simulink model "Copy_3_of_soft_switch_new_simulation"  (R2025b)
settings: Solver=ode23s  StartTime=0.0  StopTime=1  MaxStep=1e-6  RelTol=1e-5
InitFcn:
  | run param_file.m
values from neighbouring files (symbols this model uses):
  param = struct()    [Copy_of_param_file.m]    (also in param_file.m; param_file_loss_vs_freq.m; param_file_original.m; param_file_turbine.m)
settings Model: Creator=user  LastModifiedBy=user
settings SolverCC: ZeroCrossAlgorithm=Adaptive
settings DebuggingCC: IgnoredZcDiagnostic=none

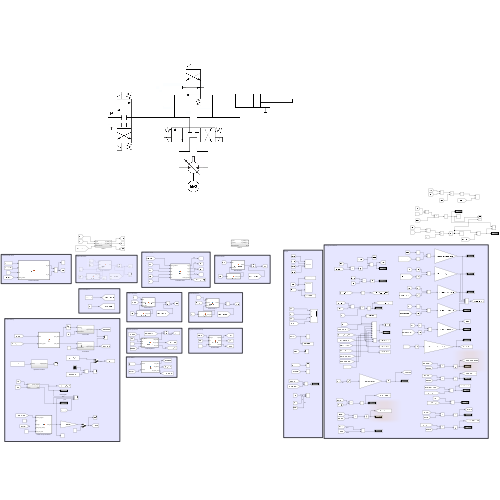
[thumbnail: Simulink's stored preview of the top-level diagram]
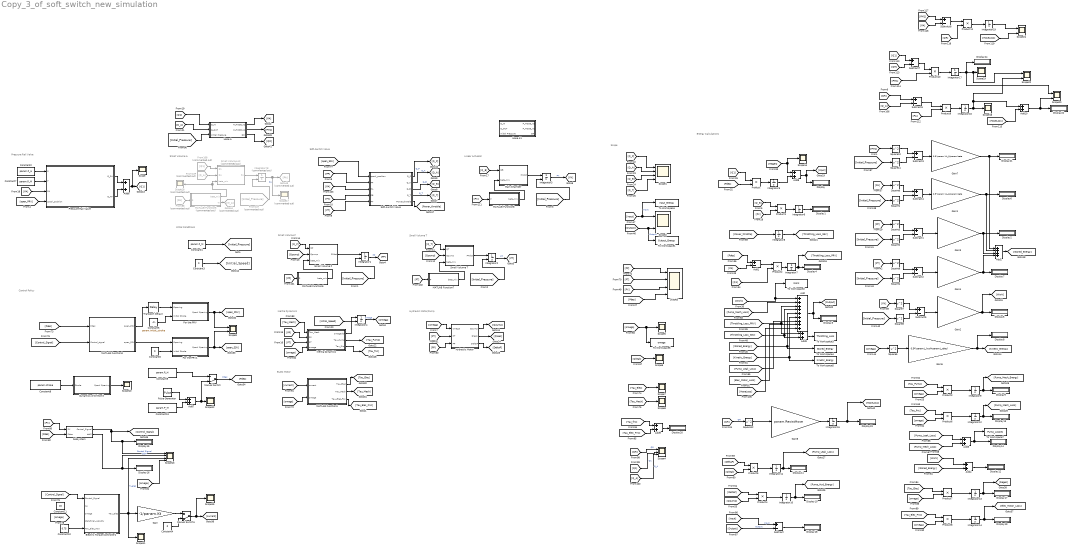
== system Copy_3_of_soft_switch_new_simulation ==
  note: Small Volume A
  note: Control Policy
  note: BLDC Motor
  note: Energy Calculations
  note: Pressure Rail Valve
  note: Scope
  note: Initial Conditions
  note: Hydraulic Motor/Pump
  note: Inertia Dynamics
  note: Small Volume T
  note: Small Volume P
  note: Soft-Switch Valve
  note: Linear Actuator
  Add : Sum  Inputs=+++++++++
  Add1 : Sum  Inputs=+-
  Add{3..10} (8 alike) : Sum
  Add2 : Sum  Inputs=++++
  Constant1 : Constant  Value=param.P_M
  Constant10 : Constant  Value=0.75
  Constant11 : Constant  Value=15
  Constant13 : Constant  Value=param.P_M
  Constant2 : Constant  Value=param.P_H
  Constant3 : Constant  Value=0
  Constant4 : Constant  Value=0
  Constant5 : Constant  Value=param.initial_stroke
  Constant6 : Constant  Value=0
  Constant7 : Constant  Value=param.P_M
  Constant8 : Constant  Value=param.stroke
  Constant9 : Constant  Value=param.P_H
  Display{,1..24} (25 alike) : Display
  Dynamics of Orifice 3 : Subsystem
  Electric Torque Controller1 : MATLAB Function  TreatAsAtomicUnit=on
  For the PRV : Subsystem
  For the PRV1 : Subsystem
  From107 : From  Commented=on  GotoTag=Initial_Pressure
  From108 : From  Commented=on  GotoTag=Q1
  From109 : From  Commented=on  GotoTag=Q_A
  From88 : From  Commented=on  GotoTag=PA
  Gain : Gain  Gain=-1/param.Kt
  Gain1 : Gain  Gain=0.5*param.VA_0/param.beta
  Gain2 : Gain  Gain=0.5*param.V1_0/param.beta
  Gain3 : Gain  Gain=0.5*param.VP_0/param.beta
  Gain4 : Gain  Gain=0.5*param.VT_0/param.beta
  Gain5 : Gain  Gain=0.5*(param.J_hyd+param.J_elec)
  Gain7 : Gain  Gain=0.5*param.VA_0/param.beta
  Gain8 : Gain  Gain=param.ResistHose
  Goto43 : Goto  Commented=on  GotoTag=PA
  Goto44 : Goto  Commented=on  GotoTag=W_A
  Hose A : Subsystem
  Hose A1 : Subsystem
  Hydraulic Motor : MATLAB Function  TreatAsAtomicUnit=on
  Inertia Dynamics : MATLAB Function  TreatAsAtomicUnit=on
  Integrator{1..4} (4 alike) : Integrator  InitialConditionSource=external
  Integrator{5..17,19} (14 alike) : Integrator
  Integrator18 : Integrator  Commented=on  InitialConditionSource=external
  MATLAB Function1 : MATLAB Function  TreatAsAtomicUnit=on
  MATLAB Function3 : MATLAB Function  TreatAsAtomicUnit=on
  MATLAB Function5 : MATLAB Function  Commented=on  TreatAsAtomicUnit=on
  MATLAB Function6 : MATLAB Function  TreatAsAtomicUnit=on
  MATLAB Function7 : MATLAB Function  TreatAsAtomicUnit=on
  MATLAB Function8 : MATLAB Function  TreatAsAtomicUnit=on
  Main Chamber : MATLAB Function  TreatAsAtomicUnit=on
  Manual Switch : ManualSwitch  CurrentSetting=0
  Manual Switch1 : ManualSwitch  CurrentSetting=0
  Pressure Rail Valve : MATLAB Function  TreatAsAtomicUnit=on
  Product{,1..11} (12 alike) : Product
  Pulse Generator : DiscretePulseGenerator  PulseType=Time based  Amplitude=param.P_H-param.P_M  Period=1.0  PulseWidth=50  PhaseDelay=param.delay
  Scope{,5..8,10..12,14..16,19} (12 alike) : Scope
      Scope settings: ActiveDisplayYMinimum=-7.8990948168927051E-6  ActiveDisplayYMaximum=6.46174239346027E-5  DataLoggingVariableName=ScopeData14
      Scope10 settings: ActiveDisplayYMinimum=-0.00062  ActiveDisplayYMaximum=0.00562  DataLoggingVariableName=ScopeData9
      Scope11 settings: ActiveDisplayYMinimum=-0.9375  ActiveDisplayYMaximum=0.9375  DataLoggingVariableName=ScopeData10
      Scope12 settings: ActiveDisplayYMinimum=2.585125E+6  ActiveDisplayYMaximum=1.1203875E+7  DataLoggingVariableName=ScopeData11
      Scope14 settings: ActiveDisplayYMinimum=-0.0475518283401892  ActiveDisplayYMaximum=0.42796645506170294  DataLoggingVariableName=ScopeData13
      Scope15 settings: ActiveDisplayYMinimum=-1  ActiveDisplayYMaximum=1  DataLoggingVariableName=ScopeData15
      Scope16 settings: ActiveDisplayYMinimum=-0.0475518283401892  ActiveDisplayYMaximum=0.42796645506170294  DataLoggingVariableName=ScopeData16
      Scope19 settings: ActiveDisplayYMinimum=-0.0475518283401892  ActiveDisplayYMaximum=0.42796645506170294  DataLoggingVariableName=ScopeData19
      Scope5 settings: ActiveDisplayYMinimum=-11.518295379628592  ActiveDisplayYMaximum=103.66465841665735  DataLoggingVariableName=ScopeData3
      Scope6 settings: ActiveDisplayYMinimum=-2.1163885820684094E-7  ActiveDisplayYMaximum=1.4152197079471591E-6  DataLoggingVariableName=ScopeData5
      Scope7 settings: ActiveDisplayYMinimum=-0.75527710182478136  ActiveDisplayYMaximum=-0.74781146844223478  DataLoggingVariableName=ScopeData6
      Scope8 settings: ActiveDisplayYMinimum=-0.030512320140982374  ActiveDisplayYMaximum=0.010920175405050834  DataLoggingVariableName=ScopeData7
  Scope1 : Scope  NumInputPorts=4
      settings: ActiveDisplayYMinimum=-0.00094060960760663083  ActiveDisplayYMaximum=0.00094060960760663083
  Scope13 : Scope  NumInputPorts=4
      settings: ActiveDisplayYMinimum=-0.12499999999999997  ActiveDisplayYMaximum=1.125  DataLoggingVariableName=ScopeData12
  Scope17 : Scope  Commented=on
      settings: ActiveDisplayYMinimum=2.181490968537122E+6  ActiveDisplayYMaximum=1.1231186415855616E+7  DataLoggingVariableName=ScopeData17
  Scope18 : Scope  Commented=on
      settings: ActiveDisplayYMinimum=1.7999999999999995E+9  ActiveDisplayYMaximum=1.8000000000000005E+9  DataLoggingVariableName=ScopeData18
  Scope{2,9,20..22} (5 alike) : Scope  NumInputPorts=2
      Scope2 settings: ActiveDisplayYMinimum=7.1801109176993929  ActiveDisplayYMaximum=9.674075574850372
      Scope20 settings: ActiveDisplayYMinimum=-0.032471059500060594  ActiveDisplayYMaximum=0.29223953550054538  DataLoggingVariableName=ScopeData20
      Scope21 settings: ActiveDisplayYMinimum=0.0065545365795663139  ActiveDisplayYMaximum=0.0079304272883429627  DataLoggingVariableName=ScopeData21
      Scope22 settings: ActiveDisplayYMinimum=-0.033093611834101345  ActiveDisplayYMaximum=0.29784250650691219  DataLoggingVariableName=ScopeData22
      Scope9 settings: ActiveDisplayYMinimum=-1.2499999999999898  ActiveDisplayYMaximum=1.2499999999999079  DataLoggingVariableName=ScopeData8
  Scope3 : Scope  NumInputPorts=4
      settings: ActiveDisplayYMinimum=-38180.936985161854  ActiveDisplayYMaximum=1.3423951077997142E+7  DataLoggingVariableName=ScopeData2
  Scope4 : Scope  NumInputPorts=3
      settings: ActiveDisplayYMinimum=-1.8027015658563681E-5  ActiveDisplayYMaximum=0.00016224314092707316  DataLoggingVariableName=ScopeData4
  Small Volume A2 : MATLAB Function  Commented=on  TreatAsAtomicUnit=on
  Small Volume P : MATLAB Function  TreatAsAtomicUnit=on
  Small Volume T : MATLAB Function  TreatAsAtomicUnit=on
  Soft-switch Valve : MATLAB Function  TreatAsAtomicUnit=on
  Square{1..12} (12 alike) : Math  Operator=square
  Subsystem : Subsystem
  Subtract{,1..8} (9 alike) : Sum  Inputs=+-
  To Workspace : ToWorkspace  VariableName=Input_Energy  SaveFormat=Timeseries  SampleTime=-1
  To Workspace1 : ToWorkspace  VariableName=Output_Energy  SaveFormat=Timeseries  SampleTime=-1
  To Workspace2 : ToWorkspace  VariableName=Work  SaveFormat=Timeseries  SampleTime=-1
  To Workspace3 : ToWorkspace  VariableName=Throttling_Loss  SaveFormat=Timeseries  SampleTime=-1
  To Workspace4 : ToWorkspace  VariableName=Stored_Energy  SaveFormat=Timeseries  SampleTime=-1
  To Workspace5 : ToWorkspace  VariableName=Kinetic_Energy  SaveFormat=Timeseries  SampleTime=-1
  To Workspace6 : ToWorkspace  VariableName=omega  SaveFormat=Timeseries  SampleTime=-1
  To Workspace7 : ToWorkspace  VariableName=Pump_Losses  SaveFormat=Timeseries  SampleTime=-1
  Transport Delay2 : TransportDelay  DelayTime=10e-3  InitialOutput=param.initial_stroke  BufferSize=1024*105
  wires:
  Constant2/1 -> Pressure Rail Valve/1(P)
  Constant1/1 -> [Initial_Pressure]
  Small Volume P/1(PPdot) -> Integrator1/1
  [Initial_Pressure] -> Integrator1/2
  Small Volume T/1(PTdot) -> Integrator2/1
  [Initial_Pressure] -> Integrator2/2
  Main Chamber/1(PXdot) -> Integrator3/1
  [Initial_Pressure] -> Integrator3/2
  Integrator3/1 -> [PX]  "PX"
  [PA] -> Soft-switch Valve/3(PA)
  [omega] -> Hydraulic Motor/1(omega)
  Integrator1/1 -> [PP]  "PP"
  Integrator2/1 -> [PT]  "PT"
  [PP] -> Soft-switch Valve/2(PP)
  [PT] -> Soft-switch Valve/5(PT)
  [PX] -> Soft-switch Valve/4(PB)
  Soft-switch Valve/4(Q_T) -> [Q_T]  "Q_T"
  Soft-switch Valve/3(Q_B) -> [Q_B]  "Q_B"
  Soft-switch Valve/2(Q_A) -> [Q_A]  "Q_A"
  [Q_T] -> Small Volume T/1(QT)
  Hydraulic Motor/1(Qpump) -> [Qpump]
  [Qpump] -> Small Volume T/2(Qpump)
  [Qpump] -> Small Volume P/2(Qpump)
  [Q_P] -> Small Volume P/1(QP)
  [Q_B] -> Main Chamber/1(QB)
  Constant3/1 -> [Initial_Speed]
  [Q_P] -> Scope1/1
  [Q_A] -> Scope1/2
  [Q_B] -> Scope1/3
  [Q_T] -> Scope1/4
  [Q1] -> Product/1
  [Pdes] -> Product/2
  Product/1 -> Integrator5/1
  [Q_B] -> Product1/1
  [PX] -> Product1/2
  Product1/1 -> Integrator6/1
  Integrator6/1 -> Display1/1
  [Work] -> To Workspace2/1, Add/1
  [Kinetic_Energy] -> To Workspace5/1, Add/6
  Add/1 -> [Output], Display3/1
  [PA] -> Add1/2
  Add1/1 -> Product2/1
  [Q1] -> Product2/2
  Product2/1 -> Integrator7/1
  Integrator7/1 -> [Throttling_Loss_PRV], Display4/1
  [Throttling_Loss_PRV] -> Add3/1, Add/3
  Soft-switch Valve/1(Q_P) -> [Q_P]  "Q_P"
  Soft-switch Valve/5(Power_throttle) -> [Power_throttle]
  [PA] -> Square6/1
  Subtract5/1 -> Gain2/1
  Gain2/1 -> [Work], Display5/1
  Gain1/1 -> Add2/2, Display6/1
  Gain3/1 -> Add2/3, Display2/1
  Gain5/1 -> Display8/1, [Kinetic_Energy]
  Square5/1 -> Gain5/1
  [omega] -> Square5/1
  [Stored_Energy] -> To Workspace4/1, Add/5
  [Initial_Pressure] -> Square1/1
  Square6/1 -> Subtract4/1
  Square1/1 -> Subtract4/2
  [PX] -> Square7/1
  [Initial_Pressure] -> Square8/1
  Subtract4/1 -> Gain1/1
  Square7/1 -> Subtract5/1
  Square8/1 -> Subtract5/2
  Square2/1 -> Subtract1/2
  Square3/1 -> Subtract1/1
  Square9/1 -> Subtract2/1
  Square4/1 -> Subtract2/2
  Subtract2/1 -> Gain4/1
  [PT] -> Square9/1
  [Initial_Pressure] -> Square4/1
  [PP] -> Square3/1
  [Initial_Pressure] -> Square2/1
  Subtract1/1 -> Gain3/1
  Gain4/1 -> Add2/4, Display7/1
  Add2/1 -> [Stored_Energy]
  [Input] -> Scope2/1, To Workspace/1  "Input"
  [Output] -> To Workspace1/1, Scope2/2  "Output"
  Integrator8/1 -> [Throttling_Loss_SSV]
  [Throttling_Loss_SSV] -> Add3/2, Add/4
  Add3/1 -> To Workspace3/1
  [PX] -> Scope3/3
  [PT] -> Inertia Dynamics/3(PT)
  Inertia Dynamics/2(Tau_Pump) -> [Tau_Pump]
  [PP] -> Inertia Dynamics/2(PP)
  [omega] -> Product3/2
  [Tau_Pump] -> Product3/1
  Integrator9/1 -> [Pump_Mech_Energy], Display9/1
  Product3/1 -> Integrator9/1
  Hydraulic Motor/3(DeltaP) -> [DeltaP]
  [DeltaP] -> Product4/1
  [Qpump] -> Product4/2
  Product4/1 -> Integrator10/1
  Integrator10/1 -> [Pump_Hyd_Energy], Display10/1
  [omega] -> To Workspace6/1, Scope5/1
  Hydraulic Motor/2(Qleak) -> [Qleak]
  [Qleak] -> Scope6/1
  [PT] -> Hydraulic Motor/2(PT)
  [PP] -> Hydraulic Motor/3(PP)
  [DeltaP] -> Product5/1
  [Qleak] -> Product5/2
  Product5/1 -> Integrator11/1
  Integrator11/1 -> [Pump_Leak_Loss], Display11/1
  [Pump_Mech_Loss] -> Add/2
  [omega] -> Inertia Dynamics/4(omega)
  Inertia Dynamics/3(Tau_Fric) -> [Tau_fric]
  [Tau_fric] -> Product6/1
  [omega] -> Product6/2
  Product6/1 -> Integrator12/1
  Integrator12/1 -> [Pump_Mech_Loss], Display13/1
  [Pump_Leak_Loss] -> Add/7
  [Pump_Leak_Loss] -> Add5/1
  [Pump_Mech_Loss] -> Add5/2
  Add5/1 -> To Workspace7/1, Display14/1
  [Work] -> Add4/1
  [Stored_Energy] -> Add4/2
  Add4/1 -> Display12/1
  [Pdes] -> Scope3/4
  [PT] -> Scope3/2
  [PP] -> Scope3/1
  [omega] -> MATLAB Function1/2(omega)
  [current] -> MATLAB Function1/1(current)
  MATLAB Function1/1(Tau_Elec) -> [Tau_Elec]
  MATLAB Function1/2(Tau_Mech) -> [Tau_Mech]
  [Tau_Elec] -> Scope7/1
  [Tau_Mech] -> Scope8/1
  For the PRV/1(Spool Opening) -> [open_PRV], Scope9/1
  For the PRV1/1(Spool Opening) -> Scope9/2, [open_SSV]
  [Control_Signal] -> MATLAB Function3/2(Control_signal)
  Transport Delay2/1 -> For the PRV/1(Opening)
  MATLAB Function3/1(open_PRV) -> Transport Delay2/1
  MATLAB Function3/2(open_SSV) -> For the PRV1/1(Opening)
  Pressure Rail Valve/1(Q_PA) -> Add6/1
  Pressure Rail Valve/2(Q_AT) -> Add6/2
  Add6/1 -> Scope/1, [Q1]
  [PA] -> Pressure Rail Valve/3(PA)
  Constant7/1 -> Pressure Rail Valve/2(T)
  [open_PRV] -> Pressure Rail Valve/4(spool_position)
  [open_SSV] -> Soft-switch Valve/1(spool_position)
  [Pdes] -> Subsystem/2(Pdes)
  [PX] -> Subsystem/1(PX)
  Subsystem/1(Control_Signal) -> [Control_Signal], Scope13/1, Display15/1  "Control Signal"
  Subsystem/2(delP) -> Scope13/2, Display16/1  "delP"
  Manual Switch/1 -> [Pdes]  "Pdes"
  Constant10/1 -> Electric Torque Controller1/5(Tau_elec_max)
  Constant9/1 -> Manual Switch/1
  Constant13/1 -> Add7/2
  Pulse Generator/1 -> Add7/1
  Add7/1 -> Manual Switch/2, Scope12/1
  Dynamics of Orifice 3/1(Spool Opening) -> Scope10/1
  Constant8/1 -> Dynamics of Orifice 3/1(Stroke)
  [omega] -> Scope13/4
  [Control_Signal] -> Electric Torque Controller1/1(Control_Signal)
  Electric Torque Controller1/1(Tau_elec) -> Gain/1, Scope13/3, Scope11/1  "T_elec"
  [Pdes] -> MATLAB Function3/1(Pdes)
  [Tau_Elec] -> Product7/1
  [omega] -> Product7/2
  Product7/1 -> Integrator13/1
  Integrator13/1 -> [Regen], Display17/1
  [Input] -> Subtract/1  "Input"
  [Output] -> Subtract/2  "Output"
  Subtract/1 -> Display18/1
  MATLAB Function1/3(Tau_Elec_Fric) -> [Tau_Elec_Fric]
  [Tau_Elec_Fric] -> Product8/1
  [omega] -> Product8/2
  Product8/1 -> Integrator14/1
  Integrator14/1 -> [Elec_Motor_Loss], Display19/1
  [Power_throttle] -> Integrator8/1
  [Pdes] -> Add1/1
  [Regen] -> Add8/1, Scope14/1
  Integrator5/1 -> Add8/2
  Add8/1 -> Display/1, [Input]
  [Tau_Mech] -> Inertia Dynamics/1(Tau_Mech)
  [Elec_Motor_Loss] -> Add/8
  [Initial_Speed] -> Integrator4/2
  Inertia Dynamics/1(omegadot) -> Integrator4/1
  Integrator4/1 -> [omega]  "omega"
  Gain/1 -> Manual Switch1/1
  Constant4/1 -> Manual Switch1/2
  Manual Switch1/1 -> Scope15/1, [current]
  [Tau_Elec_Fric] -> Add9/2
  [Tau_fric] -> Add9/1
  Add9/1 -> Display20/1
  Constant5/1 -> For the PRV/2(Initial Stroke)
  Constant6/1 -> For the PRV1/2(Initial Stroke)
  From108/1 -> Small Volume A2/1(Q1)
  From109/1 -> Small Volume A2/2(QA)
  Integrator18/1 -> Goto43/1, Scope17/1  "PA"
  From107/1 -> Integrator18/2
  Small Volume A2/1(PA) -> Integrator18/1
  MATLAB Function5/1(beta_mix) -> Small Volume A2/3(beta_mix), Scope18/1
  From88/1 -> MATLAB Function5/1(P)
  [PP] -> MATLAB Function6/1(P)
  MATLAB Function6/1(beta_mix) -> Small Volume P/3(beta_mix)
  [PT] -> MATLAB Function7/1(P)
  MATLAB Function7/1(beta_mix) -> Small Volume T/3(beta_mix)
  MATLAB Function8/1(beta_mix) -> Main Chamber/2(beta_mix)
  [PX] -> MATLAB Function8/1(P)
  MATLAB Function5/2(W) -> Goto44/1
  [Q1] -> Hose A/1(Q_IN)
  [Q_A] -> Hose A/2(Q_OUT)
  [Initial_Pressure] -> Hose A/3(Initial Pressure)
  Hose A/1(P_HOSE_V2) -> [PA]
  Hose A/2(P_HOSE_V1) -> [PM1]
  [PM1] -> Square10/1
  [Initial_Pressure] -> Square11/1
  Square10/1 -> Subtract3/1
  Square11/1 -> Subtract3/2
  Subtract3/1 -> Gain7/1
  Gain7/1 -> Add2/1, Display21/1
  Hose A/3(QR) -> [QR]
  [QR] -> Scope4/1  "QR"
  [Q1] -> Scope4/2  "Q1"
  [Q_A] -> Scope4/3  "Q_A"
  [QR] -> Square12/1  "QR"
  Square12/1 -> Gain8/1
  Gain8/1 -> Integrator15/1
  [HoseLoss] -> Add/9
  Integrator15/1 -> [HoseLoss], Display23/1
  [QR] -> Subtract6/1
  [Q_A] -> Subtract6/2
  Subtract6/1 -> Product9/1
  [PA] -> Product9/2
  Product9/1 -> Integrator16/1
  Integrator16/1 -> Add10/1, Scope22/2, Scope16/1
  [Q1] -> Subtract7/1
  [QR] -> Subtract7/2
  Subtract7/1 -> Product10/1
  [PM1] -> Product10/2
  Product10/1 -> Integrator17/1
  Integrator17/1 -> Scope20/1, Scope22/1, Scope19/1, Display24/1
  [HoseLoss] -> Add10/2
  Add10/1 -> Display22/1, Scope20/2
  Subtract8/1 -> Product11/1
  [QR] -> Product11/2
  Product11/1 -> Integrator19/1
  [HoseLoss] -> Scope21/2
  Integrator19/1 -> Scope21/1
  [PM1] -> Subtract8/1
  [PA] -> Subtract8/2

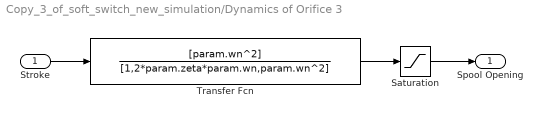
== system Copy_3_of_soft_switch_new_simulation/Dynamics of Orifice 3 ==
  Stroke : Inport
  Saturation : Saturate  UpperLimit=param.stroke  LowerLimit=0
  Transfer Fcn : TransferFcn  Numerator=[param.wn^2]  Denominator=[1,2*param.zeta*param.wn,param.wn^2]
  Spool Opening : Outport
  wires:
  Transfer Fcn/1 -> Saturation/1
  Saturation/1 -> Spool Opening/1
  Stroke/1 -> Transfer Fcn/1

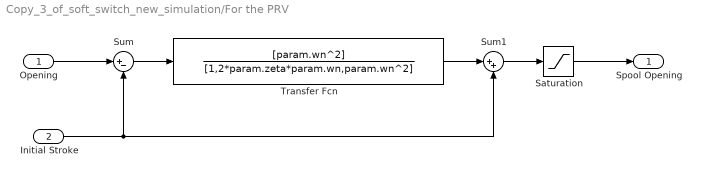
== system Copy_3_of_soft_switch_new_simulation/For the PRV ==
  Opening : Inport
  Initial Stroke : Inport  Port=2
  Saturation : Saturate  UpperLimit=1  LowerLimit=-1
  Sum : Sum  Inputs=|+-
  Sum1 : Sum  Inputs=|++
  Transfer Fcn : TransferFcn  Numerator=[param.wn^2]  Denominator=[1,2*param.zeta*param.wn,param.wn^2]
  Spool Opening : Outport
  wires:
  Saturation/1 -> Spool Opening/1
  Sum1/1 -> Saturation/1
  Transfer Fcn/1 -> Sum1/1
  Sum/1 -> Transfer Fcn/1
  Opening/1 -> Sum/1
  Initial Stroke/1 -> Sum1/2, Sum/2

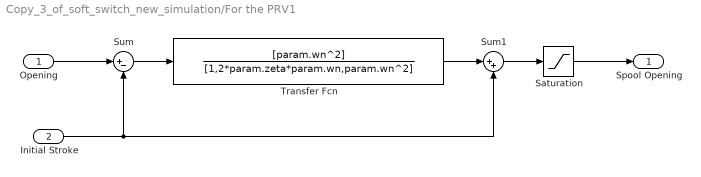
== system Copy_3_of_soft_switch_new_simulation/For the PRV1 ==
  Opening : Inport
  Initial Stroke : Inport  Port=2
  Saturation : Saturate  UpperLimit=1  LowerLimit=-1
  Sum : Sum  Inputs=|+-
  Sum1 : Sum  Inputs=|++
  Transfer Fcn : TransferFcn  Numerator=[param.wn^2]  Denominator=[1,2*param.zeta*param.wn,param.wn^2]
  Spool Opening : Outport
  wires:
  Saturation/1 -> Spool Opening/1
  Sum1/1 -> Saturation/1
  Transfer Fcn/1 -> Sum1/1
  Sum/1 -> Transfer Fcn/1
  Opening/1 -> Sum/1
  Initial Stroke/1 -> Sum1/2, Sum/2

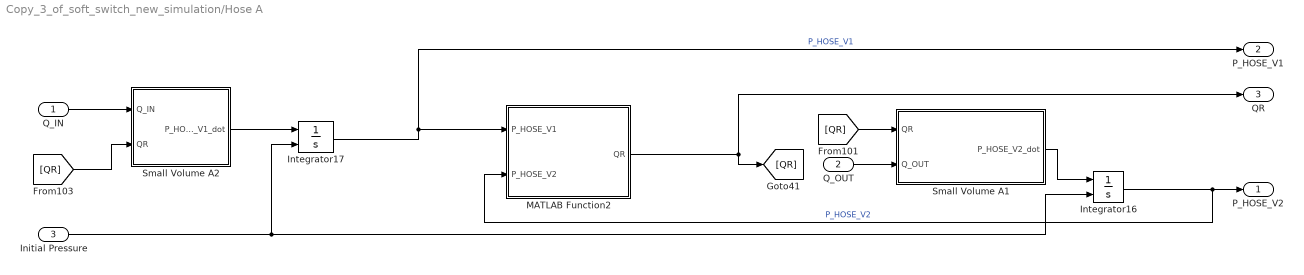
== system Copy_3_of_soft_switch_new_simulation/Hose A ==
  Q_IN : Inport
  Q_OUT : Inport  Port=2
  Initial Pressure : Inport  Port=3
  Integrator16 : Integrator  InitialConditionSource=external
  Integrator17 : Integrator  InitialConditionSource=external
  MATLAB Function2 : MATLAB Function  TreatAsAtomicUnit=on
  Small Volume A1 : MATLAB Function  TreatAsAtomicUnit=on
  Small Volume A2 : MATLAB Function  TreatAsAtomicUnit=on
  P_HOSE_V2 : Outport
  P_HOSE_V1 : Outport  Port=2
  QR : Outport  Port=3
  wires:
  Small Volume A1/1(P_HOSE_V2_dot) -> Integrator16/1
  Small Volume A2/1(P_HOSE_V1_dot) -> Integrator17/1
  MATLAB Function2/1(QR) -> [QR], QR/1
  Integrator17/1 -> MATLAB Function2/1(P_HOSE_V1), P_HOSE_V1/1  "P_HOSE_V1"
  Initial Pressure/1 -> Integrator17/2, Integrator16/2
  Q_OUT/1 -> Small Volume A1/2(Q_OUT)
  [QR] -> Small Volume A1/1(QR)
  [QR] -> Small Volume A2/2(QR)
  Integrator16/1 -> P_HOSE_V2/1, MATLAB Function2/2(P_HOSE_V2)  "P_HOSE_V2"
  Q_IN/1 -> Small Volume A2/1(Q_IN)

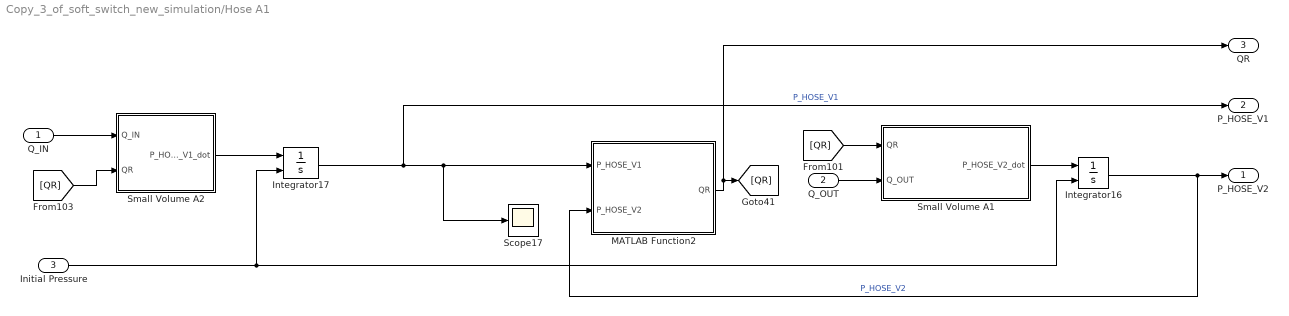
== system Copy_3_of_soft_switch_new_simulation/Hose A1 ==
  Q_IN : Inport
  Q_OUT : Inport  Port=2
  Initial Pressure : Inport  Port=3
  Integrator16 : Integrator  InitialConditionSource=external
  Integrator17 : Integrator  InitialConditionSource=external
  MATLAB Function2 : MATLAB Function  TreatAsAtomicUnit=on
  Scope17 : Scope
      settings: ActiveDisplayYMinimum=2.181490968537122E+6  ActiveDisplayYMaximum=1.1231186415855616E+7  DataLoggingVariableName=ScopeData17
  Small Volume A1 : MATLAB Function  TreatAsAtomicUnit=on
  Small Volume A2 : MATLAB Function  TreatAsAtomicUnit=on
  P_HOSE_V2 : Outport
  P_HOSE_V1 : Outport  Port=2
  QR : Outport  Port=3
  wires:
  Q_IN/1 -> Small Volume A2/1(Q_IN)
  Integrator16/1 -> P_HOSE_V2/1, MATLAB Function2/2(P_HOSE_V2)  "P_HOSE_V2"
  [QR] -> Small Volume A2/2(QR)
  [QR] -> Small Volume A1/1(QR)
  Q_OUT/1 -> Small Volume A1/2(Q_OUT)
  Initial Pressure/1 -> Integrator16/2, Integrator17/2
  Integrator17/1 -> P_HOSE_V1/1, Scope17/1, MATLAB Function2/1(P_HOSE_V1)  "P_HOSE_V1"
  MATLAB Function2/1(QR) -> [QR], QR/1
  Small Volume A2/1(P_HOSE_V1_dot) -> Integrator17/1
  Small Volume A1/1(P_HOSE_V2_dot) -> Integrator16/1

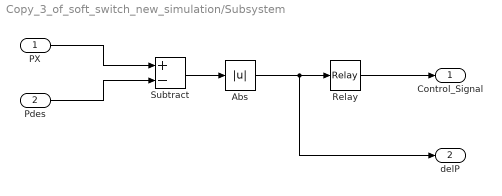
== system Copy_3_of_soft_switch_new_simulation/Subsystem ==
  PX : Inport
  Pdes : Inport  Port=2
  Abs : Abs  SaturateOnIntegerOverflow=off
  Relay : Relay  OnSwitchValue=6e5  OffSwitchValue=1e4  OnOutputValue=0  OffOutputValue=1
  Subtract : Sum  Inputs=+-
  Control_Signal : Outport
  delP : Outport  Port=2
  wires:
  PX/1 -> Subtract/1
  Pdes/1 -> Subtract/2
  Subtract/1 -> Abs/1
  Abs/1 -> delP/1, Relay/1
  Relay/1 -> Control_Signal/1

== matlab function Copy_3_of_soft_switch_new_simulation/MATLAB Function3 ==
  data: Pdes input; open_PRV output; open_SSV output; param parameter; Control_signal input
function [open_PRV, open_SSV] = fcn(Pdes, param, Control_signal)

if Pdes == param.P_H && Control_signal == 0
    open_PRV = 1;
    open_SSV = 1;

elseif Pdes == param.P_M && Control_signal == 0
    open_PRV = -1;
    open_SSV = -1;

elseif Pdes == param.P_H && Control_signal > 0
    open_PRV = 1;
    open_SSV = 0;

elseif Pdes == param.P_M && Control_signal > 0
    open_PRV = -1;
    open_SSV = 0;
    
else
    open_PRV = 0;
    open_SSV = 0;
end

== matlab function Copy_3_of_soft_switch_new_simulation/Hose A1/Small Volume A1 ==
  data: QR input; P_HOSE_V2_dot output; Q_OUT input; param parameter
function P_HOSE_V2_dot = Small_Vol_A(QR, Q_OUT, param)

P_HOSE_V2_dot = (param.beta/param.VA_0) * (QR - Q_OUT);

end

== matlab function Copy_3_of_soft_switch_new_simulation/MATLAB Function1 ==
  data: current input; omega input; Tau_Elec output; param parameter; Tau_Mech output; Tau_Elec_Fric output
function [Tau_Elec, Tau_Mech, Tau_Elec_Fric] = BLDC(current, omega, param)

% Limit current to stall current
I_stall = 69;
current = min(max(current, -I_stall), I_stall);

% Electromagnetic torque
Tau_Elec = param.Kt * current;

% Friction torque (viscous model)
Tau_Elec_Fric = param.B * omega;

% Mechanical torque available at shaft
Tau_Mech = Tau_Elec - Tau_Elec_Fric;

end

== matlab function Copy_3_of_soft_switch_new_simulation/Hose A/Small Volume A1 ==
  data: QR input; P_HOSE_V2_dot output; Q_OUT input; param parameter
function P_HOSE_V2_dot = Small_Vol_A(QR, Q_OUT, param)

P_HOSE_V2_dot = (param.beta/param.VA_0) * (QR - Q_OUT);

end

== matlab function Copy_3_of_soft_switch_new_simulation/Electric Torque Controller1 ==
  data: Control_Signal input; Kp input; omega input; Tau_elec output; start_final_velocity input; Tau_elec_max input
function Tau_elec  = fcn(Control_Signal, Kp, omega, start_final_velocity, Tau_elec_max)

if Control_Signal == 1 
   Tau_elec = -Tau_elec_max;
else
   Tau_elec = Tau_elec_max;
end

== matlab function Copy_3_of_soft_switch_new_simulation/Hose A/Small Volume A2 ==
  data: Q_IN input; P_HOSE_V1_dot output; QR input; param parameter
function P_HOSE_V1_dot = Small_Vol_M(Q_IN, QR, param)

P_HOSE_V1_dot = (param.beta/param.VA_0) * (Q_IN - QR);

end

== matlab function Copy_3_of_soft_switch_new_simulation/Hose A/MATLAB Function2 ==
  data: P_HOSE_V1 input; P_HOSE_V2 input; QR output; param parameter
function QR = Hose_Resistance(P_HOSE_V1, P_HOSE_V2, param)

QR = (P_HOSE_V1 - P_HOSE_V2) / param.ResistHose;

end

== matlab function Copy_3_of_soft_switch_new_simulation/Small Volume A2 ==
  data: Q1 input; PA output; QA input; beta_mix input; param parameter
function PA = Small_Vol_A(Q1,QA, beta_mix, param)

PA = (beta_mix/param.VA_0)*(Q1-QA);

== matlab function Copy_3_of_soft_switch_new_simulation/MATLAB Function5 ==
  data: P input; beta_mix output; param parameter; W output
function [beta_mix, W] = oil_comp(P,param)

Pg = P-param.P_T;   % Gauge pressure
r = P/param.P_T;    % Pressure ratio
e = exp(Pg/param.beta); 
rv = (1./e+param.air*r.^(-1/param.gamma))/(1+param.air);      %Volume ratio

beta_mix = rv*(1+param.air)/(1/(e*param.beta)+...
           param.air/(param.gamma*param.P_T*r^(1/param.gamma+1)));

El = param.beta*(e - (1 + Pg/param.beta)) + param.P_T*(e - 1);              % Energy in liquid
Eg = P/(param.gamma - 1) .* (1 - r.^(1/param.gamma - 1));           % Energy in gas
E  = (El./e + param.air*Eg.*r.^(-1/param.gamma)) ./ ...
     (1./e + param.air*r.^(-1/param.gamma));                       % Energy in mixture
W  = E - (1./rv - 1)*param.P_M;                                 % Compressibility energy density

== matlab function Copy_3_of_soft_switch_new_simulation/MATLAB Function6 ==
  data: P input; beta_mix output; param parameter
function beta_mix = oil_comp(P,param)

%Ph=7e6, P0=1e5
Pg = P-param.P_T;   % Gauge pressure
r = P/param.P_T;    % Pressure ratio
e = exp(Pg/param.beta); 
rv = (1./e+param.air*r.^(-1/param.gamma))/(1+param.air);      %Volume ratio

beta_mix = rv*(1+param.air)/(1/(e*param.beta)+...
           param.air/(param.gamma*param.P_T*r^(1/param.gamma+1)));

== matlab function Copy_3_of_soft_switch_new_simulation/Hose A1/MATLAB Function2 ==
  data: P_HOSE_V1 input; P_HOSE_V2 input; QR output; param parameter
function QR = Hose_Resistance(P_HOSE_V1, P_HOSE_V2, param)

QR = (P_HOSE_V1 - P_HOSE_V2) / param.ResistHose;

end

== matlab function Copy_3_of_soft_switch_new_simulation/MATLAB Function7 ==
  data: P input; beta_mix output; param parameter
function beta_mix = oil_comp(P,param)

%Ph=7e6, P0=1e5
Pg = P-param.P_T;   % Gauge pressure
r = P/param.P_T;    % Pressure ratio
e = exp(Pg/param.beta); 
rv = (1./e+param.air*r.^(-1/param.gamma))/(1+param.air);      %Volume ratio

beta_mix = rv*(1+param.air)/(1/(e*param.beta)+...
           param.air/(param.gamma*param.P_T*r^(1/param.gamma+1)));

== matlab function Copy_3_of_soft_switch_new_simulation/MATLAB Function8 ==
  data: P input; beta_mix output; param parameter
function beta_mix = oil_comp(P,param)

%Ph=7e6, P0=1e5
Pg = P-param.P_T;   % Gauge pressure
r = P/param.P_T;    % Pressure ratio
e = exp(Pg/param.beta); 
rv = (1./e+param.air*r.^(-1/param.gamma))/(1+param.air);      %Volume ratio

beta_mix = rv*(1+param.air)/(1/(e*param.beta)+...
           param.air/(param.gamma*param.P_T*r^(1/param.gamma+1)));

== matlab function Copy_3_of_soft_switch_new_simulation/Hose A1/Small Volume A2 ==
  data: Q_IN input; P_HOSE_V1_dot output; QR input; param parameter
function P_HOSE_V1_dot = Small_Vol_M(Q_IN, QR, param)

P_HOSE_V1_dot = (param.beta/param.VA_0) * (Q_IN - QR);

end

== matlab function Copy_3_of_soft_switch_new_simulation/Pressure Rail Valve ==
  data: P input; T input; Q_PA output; Q_AT output; PA input; spool_position input; param parameter
function [Q_PA, Q_AT] = RailValve(P, T, PA, spool_position, param)

db = 0.02;

spool_position = max(-1, min(1, spool_position));

if abs(spool_position) <= db
    f = 0;
else
    f = (abs(spool_position) - db) / (1 - db);
    f = max(0, min(1, f));
end

A_PA = 0;
A_AT = 0;

if spool_position > db
    A_PA = param.max_Avt * f;
elseif spool_position < -db
    A_AT = param.max_Avt * f;
end

Q_PA = param.Cd * A_PA * sqrt(2/param.rho) * sqrt(abs(P-PA)) * sign(P-PA);
Q_AT = param.Cd * A_AT * sqrt(2/param.rho) * sqrt(abs(PA-T)) * sign(T-PA);

end

== matlab function Copy_3_of_soft_switch_new_simulation/Soft-switch Valve ==
  data: spool_position input; Q_P output; PP input; PA input; PB input; PT input; Q_A output; Q_B output; Q_T output; param parameter; Power_throttle output
function [Q_P, Q_A, Q_B, Q_T, Power_throttle] = SSV(spool_position, PP, PA, PB, PT, param)

db = 0.02; % spool deadband around zero (fraction of full stroke)

spool_position = max(-1, min(1, spool_position));

if abs(spool_position) <= db
    f = 0;
else
    f = (abs(spool_position) - db) / (1 - db);
    f = max(0, min(1, f));
end

A_PA = 0; A_PB = 0; A_AT = 0; A_BT = 0; A_PT = 0; A_AB = 0;

if abs(spool_position) <= db
    A_PT = param.max_Avt;
    A_AB = param.max_Avt;
elseif spool_position > 0
    A_PA = param.max_Avt * f;
    A_BT = param.max_Avt * f;
elseif spool_position < 0
    A_PB = param.max_Avt * f;
    A_AT = param.max_Avt * f;
end

Q_PA = param.Cd*A_PA*sign(PP-PA)*sqrt((2/param.rho)*abs(PP-PA));
Q_PB = param.Cd*A_PB*sign(PP-PB)*sqrt((2/param.rho)*abs(PP-PB));
Q_AT = param.Cd*A_AT*sign(PA-PT)*sqrt((2/param.rho)*abs(PA-PT));
Q_BT = param.Cd*A_BT*sign(PB-PT)*sqrt((2/param.rho)*abs(PB-PT));
Q_PT = param.Cd*A_PT*sign(PP-PT)*sqrt((2/param.rho)*abs(PP-PT));
Q_AB = param.Cd*A_AB*sign(PA-PB)*sqrt((2/param.rho)*abs(PA-PB));

Q_P = -(Q_PA + Q_PB + Q_PT);
Q_A =  Q_AT + Q_AB - Q_PA;
Q_B =  Q_BT - Q_AB - Q_PB;
Q_T =  -Q_PT - Q_AT - Q_BT;

Q_B = -Q_B;

Power_throttle = ...
    abs(Q_PA)*abs(PP-PA) + ...
    abs(Q_PB)*abs(PP-PB) + ...
    abs(Q_AT)*abs(PA-PT) + ...
    abs(Q_BT)*abs(PB-PT) + ...
    abs(Q_PT)*abs(PP-PT) + ...
    abs(Q_AB)*abs(PA-PB);

end

== matlab function Copy_3_of_soft_switch_new_simulation/Small Volume P ==
  data: QP input; PPdot output; Qpump input; param parameter; beta_mix input
function PPdot = Small_Vol_P(QP,Qpump, param, beta_mix)

PPdot = (beta_mix/param.VP_0)*(QP-Qpump);

== matlab function Copy_3_of_soft_switch_new_simulation/Hydraulic Motor ==
  data: Qpump output; Qleak output; omega input; PT input; PP input; param parameter; DeltaP output
function [Qpump, Qleak, DeltaP] = Hyd_Motor(omega, PT, PP, param)
    % Analytical leakage model (Simscape-equivalent)
    
    % Parameters
    D     = param.D;          
    eta_v = param.eta_v_nom;  % nominal volumetric efficiency
    omega_nom = param.omega_nom;      % [rad/s]
    DeltaP_nom = param.dp_nom;    % [Pa]
    rho   = param.rho;        % [kg/m^3]
    
    % Pressure difference
    DeltaP = PP - PT;
    
    % Hagen–Poiseuille coefficient
    K = (D/(2*pi))*omega_nom*(1 - eta_v)/DeltaP_nom;
    
    % Mass leakage flow
    m_dot_leak = K * rho * DeltaP;
    
    % Convert to volumetric leakage
    Qleak = m_dot_leak / rho;
    
    % Ideal displacement flow
    Qideal = (D/(2*pi)) * omega;
    
    % Net flow (same convention as Simscape)
    Qpump = Qideal + Qleak;
end

== matlab function Copy_3_of_soft_switch_new_simulation/Small Volume T ==
  data: QT input; PTdot output; Qpump input; param parameter; beta_mix input
function PTdot = Small_Vol_T(QT,Qpump,param, beta_mix)

PTdot = (beta_mix/param.VT_0)*(Qpump-QT);

== matlab function Copy_3_of_soft_switch_new_simulation/Main Chamber ==
  data: QB input; PXdot output; param parameter; beta_mix input
function PXdot = Main_Chamber(QB, param, beta_mix)

PXdot = (param.beta/param.V1_0)*(QB);

== matlab function Copy_3_of_soft_switch_new_simulation/Inertia Dynamics ==
  data: Tau_Mech input; omegadot output; param parameter; PP input; PT input; Tau_Pump output; omega input; Tau_Fric output
function [omegadot, Tau_Pump, Tau_Fric] = Inertia_Dyn(Tau_Mech, param, PP, PT, omega)

dP = PP - PT;

Tau_Ideal = (param.D/(2*pi)) * dP;

Tau_fr_nom = ((1 - param.eta_m_nom)/param.eta_m_nom) ...
              * (param.D/(2*pi)) * param.dp_nom;

k = (Tau_fr_nom - param.tau0) / param.dp_nom;

omega_nom_rad = 2*pi*param.omega_nom/60;

s = tanh(4*omega/(5e-5*omega_nom_rad));

Tau_Fric = (param.tau0 + k*abs(dP)) * s;

Tau_Pump = Tau_Ideal - Tau_Fric;

omegadot = (Tau_Pump + Tau_Mech) / (param.J_hyd + param.J_elec);

end
